simulink model "Q11_1_SIM"  (R2024b)
settings: Solver=VariableStepAuto  StartTime=0.0  StopTime=10.0  RelTol=1e-3
values from neighbouring files (symbols this model uses):
  A_aug = [A zeros(5,1) ... (first row only)    [main.m]    (also in main_sim.m)
  B_aug = [B; 0]    [main.m]    (also in main_sim.m)
  C_aug = [C zeros(2,1)]    [main.m]    (also in main_sim.m)
  D = zeros(2,1)    [main.m]
  K_aug = lqr(A_aug, B_aug, Qr, Rr)    [main.m]
  L_aug = [L ... (first row only)    [main.m]    (also in main_sim.m)
  x0 = [alpha_init 0 beta_init 0 0]'    [main.m]    (also in main_sim.m = [alpha_init 0 beta_init 0 0])
undefined symbols (not defined in the file or in its folder): A, B, C
libraries: simulink_extras x1
settings Model: Creator=pedro  LastModifiedBy=pedro

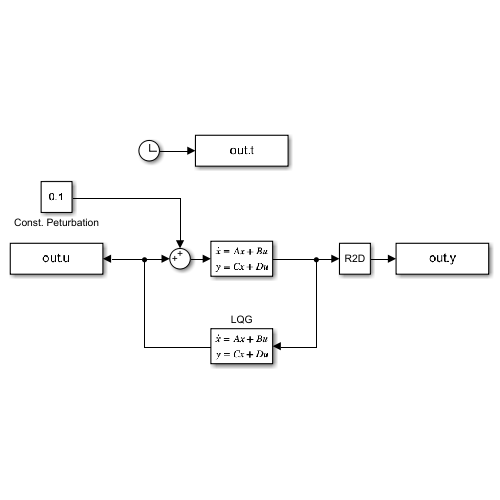
[thumbnail: Simulink's stored preview of the top-level diagram]
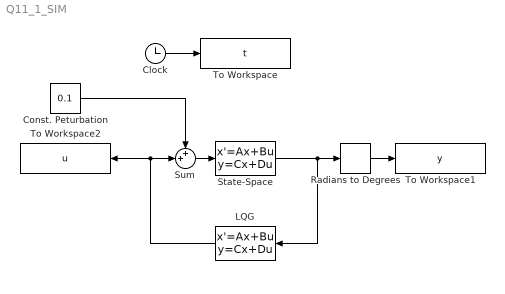
== system Q11_1_SIM ==
  Clock : Clock
  Const. Peturbation : Constant  Value=0.1
  LQG : StateSpace  A=A_aug - B_aug * K_aug - L_aug * C_aug  B=L_aug  C=-K_aug  D=zeros(1,2)  InitialCondition=0
  Radians to Degrees : simulink_extras/Transformations/Radians to Degrees
  State-Space : StateSpace  A=A  B=B  C=C  D=D  InitialCondition=x0
  Sum : Sum  Inputs=++|
  To Workspace : ToWorkspace  VariableName=t  SaveFormat=Timeseries  SampleTime=-1
  To Workspace1 : ToWorkspace  VariableName=y  SaveFormat=Timeseries  SampleTime=-1
  To Workspace2 : ToWorkspace  VariableName=u  SaveFormat=Timeseries  SampleTime=-1
  wires:
  LQG/1 -> To Workspace2/1, Sum/2
  Clock/1 -> To Workspace/1
  State-Space/1 -> Radians to Degrees/1, LQG/1
  Sum/1 -> State-Space/1
  Const. Peturbation/1 -> Sum/1
  Radians to Degrees/1 -> To Workspace1/1
